simulink model "BCIsimulink"  (R2023b)
settings: Solver=VariableStepAuto  StartTime=0.0  StopTime=10.0  RelTol=1e-3
undefined symbols (not defined in the file or in its folder): fdesignblkfcn, gcbh
settings Model: Creator=17656  LastModifiedBy=17656

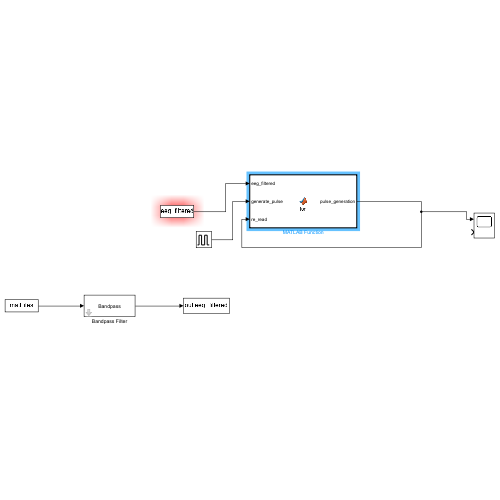
[thumbnail: Simulink's stored preview of the top-level diagram]
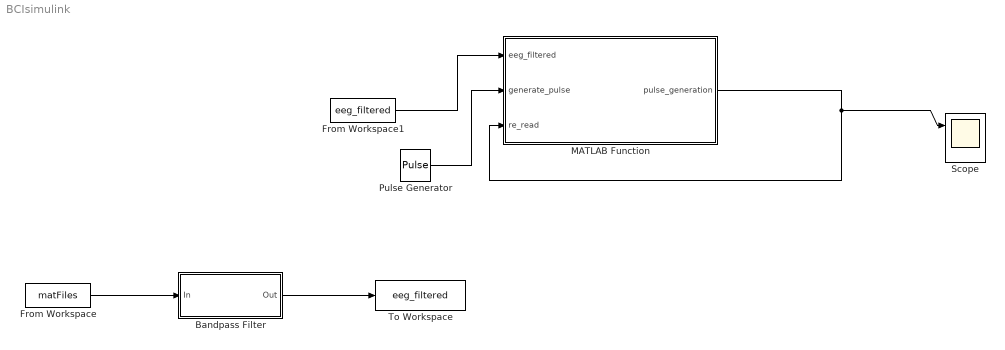
== system BCIsimulink ==
  Bandpass Filter : Subsystem  DialogController=fdesignblkfcn  InitFcn=fdesignblkfcn(gcbh, {'InitFcn'});  mask(Bandpass Filter){}
      mask help: dsp:DSPFilterDesignBlockDialog:BandpassFdesign_MaskDesc
      settings: CopyFcn=fdesignblkfcn(gcbh, {'CopyFcn'});
      mask Help: helpview(mapfilelocation('dsp'), 'dspbandpassfilter');
      mask Display: disp('Bandpass');
  From Workspace : FromWorkspace  VariableName=matFiles
  From Workspace1 : FromWorkspace  VariableName=eeg_filtered
  MATLAB Function : MATLAB Function  TreatAsAtomicUnit=on
  Pulse Generator : DiscretePulseGenerator  PulseType=Time based  Period=10  PulseWidth=5
  Scope : Scope  NumInputPorts=2
  To Workspace : ToWorkspace  VariableName=eeg_filtered  SaveFormat=Structure  SampleTime=-1
  wires:
  From Workspace/1 -> Bandpass Filter/1(In)
  Bandpass Filter/1(Out) -> To Workspace/1
  MATLAB Function/1(pulse_generation) -> MATLAB Function/3(re_read), Scope/1
  From Workspace1/1 -> MATLAB Function/1(eeg_filtered)
  Pulse Generator/1 -> MATLAB Function/2(generate_pulse)

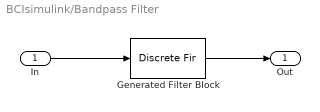
== system BCIsimulink/Bandpass Filter ==
  In : Inport
  Generated Filter Block : DiscreteFir  Tag=BlockMethodSubSystem  Coefficients=[-0.0006939392823984735 -0.000453503047195787383 -0.000554847844681304525 -0.000631227820673596293 -0.000669189870506134562 -0.00065813343723531109 -0.00059001627987731529 -0.000461764129342106123 -0.00027684141888215623 -4.53991731016917298e-05 0.000219889958781164293 0.00049670244151323983 0.000764304252813848462 0.000998819969616423359 0.00117910105157392514 0.00128857636862268038 0.00131691778026890973 0.00126152593576567967 0.00112837183240493554 0.000931906480702686998 0.000692413805193299744 0.000435933248611456619 0.000189202070639665852 -2.22450657417023936e-05 -0.000177540444433809969 -0.000263560025269521587 -0.000276281942714822241 -0.000221900683571858812 -0.000116021507587715084 1.73445612011712295e-05 0.000149696001650441609 0.000250142050285625725 0.000290655780879520349 0.000249066299251797323 0.000112762184544656224 -0.000119207191147919947 -0.000435002679001694802 -0.000810873359374447234 -0.00121303218142656296 -0.0016010760190164194 -0.0019325701762629168 -0.00216752260812475917 -0.0022732261966109538 -0.00222841411920346108 -0.00202574708611486486 -0.00167362766044916846 -0.00119538764499045646 -0.000627591885816444219 -1.59463873267743045e-05 0.000588781340535446005 0.00113683108025463544 0.00158390978200862766 0.00189640779844651324 0.00205433886513975558 0.00205346310368044243 0.00190502734227418436 0.00163438722145926038 0.00127742652536385563 0.000876480948043114076 0.000475244360068962377 0.000113969534610705537 -0.000174968831700186974 -0.000369974199197129839 -0.000462347856211100226 -0.000455895403079546789 -0.000365921897329693469 -0.000215986255290098782 -3.46689250804785428e-05 0.000149033907853164086 0.000309008245734484024 0.000425873798549258138 0.000488539435065490218 0.000495473316525877087 0.00045372129404201532 0.000377423791507386266 0.000284660345124460046 0.00019457300033039448 0.000123721616530225828 8.36273065463332028e-05 7.86218507310735507e-05 0.00010541320412368329 0.000153302132542685828 0.000206326396598760997 0.000245428729510595116 0.000252094245113707559 0.00021109263661581851 0.000113693646952601893 -4.09198819730128443e-05 -0.000244402749373046589 -0.000480390965464510991 -0.000725812147229956575 -0.000954229927923561571 -0.00113892662608551824 -0.00125692932972896652 -0.00129189816967711707 -0.00123696053614390147 -0.00109555397599958278 -0.000881632609035120436 -0.000617788826793532159 -0.000332803969632387625 -5.77027565460282144e-05 0.000177829577112486985 0.000349676970892288756 0.000441950214147924906 0.000449408520275162841 0.000377625470962871651 0.000242538351137593599 6.7747053883643858e-05 -0.000118290003259982298 -0.000286616717768329481 -0.00041127904184255613 -0.000473175916061579778 -0.000462199486112379839 -0.000378780097260280832 -0.000233268459141877692 -4.46149739228800636e-05 0.000162809001482003138 0.000362495584824324769 0.000529924359442954435 0.000645775072856247961 0.000698964075817652014 0.000687770250765850342 0.000620310322638127371 0.000512816299645163422 0.000387448526519056308 0.000268513440311248788 0.00017908246505780103 0.000137033182883509552 0.000152609685980028805 0.000226365706473455764 0.000349222022963104777 0.000503352904796189023 0.000664962386075236079 0.000807439783914938353 0.00090555614678194615 0.000938976821425020454 0.000895670417888264785 0.000773666555431560773 0.000581888934493652189 0.000338913888196190735 7.0880459828622064e-05 -0.000192327019332254009 -0.000420878093240264594 -0.000589458287834430613 -0.00068057245808801094 -0.000687363687234661186 -0.000614375452276703839 -0.000477306682186043156 -0.000300597481131130917 -0.000114303363533468851 5.03551786542749962e-05 0.000165188466750056605 0.000209285289879440736 0.000171809539739290406 5.38460739125722152e-05 -0.000131883615766872453 -0.000362535564532821407 -0.000608516570902242499 -0.000837425736966519643 -0.00101885745019053412 -0.00112847456968319165 -0.00115172378441694883 -0.0010856886815298135 -0.000939751771504392444 -0.000734041815464579707 ...(+20035 chars)]  InputProcessing=Columns as channels (frame based)
  Out : Outport  VectorParamsAs1DForOutWhenUnconnected=off
  wires:
  In/1 -> Generated Filter Block/1
  Generated Filter Block/1 -> Out/1

== matlab function BCIsimulink/MATLAB Function ==
  data: eeg_filtered input; pulse_generation output; generate_pulse input; re_read input
function pulse_generation = fcn(eeg_filtered, generate_pulse, re_read)

% Hjorth Activity, Mobility, Complexity
f1 = jfeeg('ha', X);
f2 = jfeeg('hm', X);
f3 = jfeeg('hc', X);

% Feature vector for Hjorth features
hjorth_feat = [f1, f2, f3];

% Band Power Alpha, Tsallis Entropy
opts.fs = 500;
f4 = jfeeg('bpa', X, opts);
opts.alpha = 2;
f5 = jfeeg('te', X, opts);

% Feature vector for additional features
additional_feat = [f4, f5];

% Combine all features into a single feature vector
feat = [hjorth_feat, additional_feat];

% Decide pulse generation based on extracted features
threshold_activity = 0.5; % Adjust as needed
threshold_tsallis_entropy = 0.7; % Adjust as needed

generate_pulse = (f1 > threshold_activity) && (f5 > threshold_tsallis_entropy);

% generate_pulse variable to contro pulse generator
if generate_pulse
    disp('Generate Pulse!');
    % Your code to generate a pulse at a specific frequency goes here
else
    disp('Do not generate pulse.');
    % Your code when no pulse should be generated goes here
end
